simulink model "ct_system"  (R2022a)
settings: Solver=ode45  StartTime=0.0  StopTime=tfinal  FixedStep=T  MaxStep=0.01  RelTol=1e-12  AbsTol=1e-12  EnableMultiTasking=on
values from neighbouring files (symbols this model uses):
  input_freq = (1/64)    (= 0.015625)    [lead_controller_design.m]
  k2 = 0.0609    [controllers.m]
  k3 = -4.36    [controllers.m]
  r_amp = 0.015    [lead_controller_design.m]
  r_dc_offset = 0.165    [lead_controller_design.m]
libraries: cstblocks x3
settings Model: Creator=cnielsen  LastModifiedBy=urban
settings SolverCC: AutoScaleAbsTol=off  AlgebraicLoopSolver=TrustRegion
settings DataIOCC: SaveFormat=Array  SignalLoggingSaveFormat=ModelDataLogs  SaveOutput=off  SaveTime=off  ReturnWorkspaceOutputs=off  Refine=5
settings OptimizationCC: ExpressionDepthLimit=2147483647  LifeSpan=inf
settings DebuggingCC: UnderspecifiedInitializationDetection=Classic  MergeDetectMultiDrivingBlocksExec=none  SolverPrmCheckMsg=warning  FcnCallInpInsideContextMsg=warning  UnconnectedInputMsg=warning  UnconnectedOutputMsg=warning  UnconnectedLineMsg=warning  StateNameClashWarn=warning  SFUnexpectedBacktrackingDiag=warning  SFNoUnconditionalDefaultTransitionDiag=warning  SFExecutionAtInitializationDiag=none  SFMachineParentedDataDiag=warning  ArithmeticOperatorsInVariantConditions=warning
settings HardwareCC: ProdBitPerPointer=32  ProdBitPerSizeT=32  ProdBitPerPtrDiffT=32  ProdLargestAtomicFloat=None  ProdIntDivRoundTo=Undefined  ProdEndianess=Unspecified  ProdWordSize=32  ProdHWDeviceType=32-bit Generic
settings ModelReferenceCC: PropagateSignalLabelsOutOfModel=off
settings SFSimCC: SimUseLocalCustomCode=off  CustomCodeUndefinedFunction=UseInterfaceOnly
settings RTWCC: RTWUseLocalCustomCode=off
settings CodeAppCC: StateflowObjectComments=on
settings GRTTargetCC: TargetLangStandard=C89/C90 (ANSI)  CombineOutputUpdateFcns=off  GRTInterface=on
settings ConfigComp: CovMetricSettings=dw  CovSaveCumulativeToWorkspaceVar=on  CovSaveSingleToWorkspaceVar=on  CovExternalEMLEnable=off

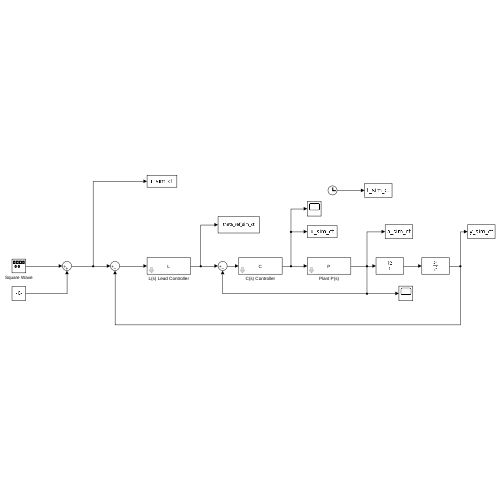
[thumbnail: Simulink's stored preview of the top-level diagram]
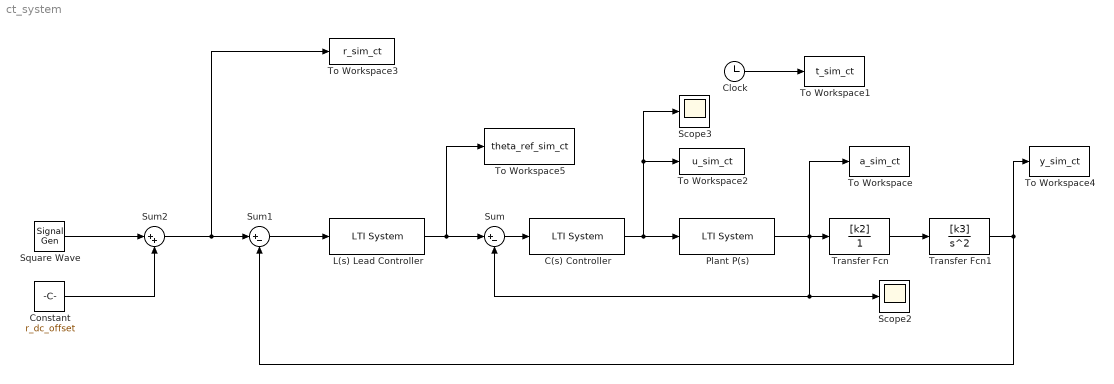
== system ct_system ==
  C(s) Controller : cstblocks/LTI System  sys=C  IC=[]
  Clock : Clock
  Constant : Constant  Value=r_dc_offset
  L(s) Lead Controller : cstblocks/LTI System  sys=L  IC=[]
  Plant P(s) : cstblocks/LTI System  sys=P  IC=[]
  Scope2 : Scope
  Scope3 : Scope
  Square Wave : SignalGenerator  WaveForm=square  Amplitude=r_amp  Frequency=input_freq
  Sum : Sum  Inputs=|+-
  Sum1 : Sum  Inputs=|+-
  Sum2 : Sum  Inputs=|++
  To Workspace : ToWorkspace  VariableName=a_sim_ct  SampleTime=-1
  To Workspace1 : ToWorkspace  VariableName=t_sim_ct  SampleTime=-1
  To Workspace2 : ToWorkspace  VariableName=u_sim_ct
  To Workspace3 : ToWorkspace  VariableName=r_sim_ct
  To Workspace4 : ToWorkspace  VariableName=y_sim_ct  SampleTime=-1
  To Workspace5 : ToWorkspace  VariableName=theta_ref_sim_ct
  Transfer Fcn : TransferFcn  Numerator=[k2]  Denominator=[0 1]
  Transfer Fcn1 : TransferFcn  Numerator=[k3]  Denominator=[1 0 0]
  wires:
  Clock/1 -> To Workspace1/1
  Plant P(s)/1 -> Transfer Fcn/1, To Workspace/1, Sum/2, Scope2/1
  C(s) Controller/1 -> Plant P(s)/1, To Workspace2/1, Scope3/1
  Sum/1 -> C(s) Controller/1
  Transfer Fcn/1 -> Transfer Fcn1/1
  Transfer Fcn1/1 -> To Workspace4/1, Sum1/2
  Sum1/1 -> L(s) Lead Controller/1
  L(s) Lead Controller/1 -> To Workspace5/1, Sum/1
  Square Wave/1 -> Sum2/1
  Sum2/1 -> To Workspace3/1, Sum1/1
  Constant/1 -> Sum2/2
